simulink model "Feedback_NearestNeighbor"  (R2015a)
settings: Solver=ode3  StartTime=0.0  StopTime=500  FixedStep=0.01  MaxStep=0.01  RelTol=1e-3
values from neighbouring files (symbols this model uses):
  H0 = interp1q(Periodic_Solution(:,1),Periodic_Solution(:,4),Initial_Time-6)    [Feedback_Nearest_Neighbour_cross_validation.m]
  Imax = 10000    [Feedback_Nearest_Neighbour_cross_validation.m]
  n0 = interp1q(Periodic_Solution(:,1),Periodic_Solution(:,7),Initial_Time-6)    [Feedback_Nearest_Neighbour_cross_validation.m]
  Periodic_Solution = Periodic_Solution(N:end,:)    [Feedback_Nearest_Neighbour_cross_validation.m]
  Sleep0 = interp1q(Periodic_Solution(:,1),Periodic_Solution(:,6),Initial_Time-6)    [Feedback_Nearest_Neighbour_cross_validation.m]
  tol = 0.01    [Feedback_Nearest_Neighbour_cross_validation.m]
  x0 = interp1q(Periodic_Solution(:,1),Periodic_Solution(:,2),Initial_Time-6)    [Feedback_Nearest_Neighbour_cross_validation.m]
  xc0 = interp1q(Periodic_Solution(:,1),Periodic_Solution(:,3),Initial_Time-6)    [Feedback_Nearest_Neighbour_cross_validation.m]
undefined symbols (not defined in the file or in its folder): Train_Sleep, Train_Wake
settings Model: Creator=wangf7  LastModifiedBy=Jiawei Yin
settings OptimizationCC: ExpressionDepthLimit=2147483647
settings DebuggingCC: AlgebraicLoopMsg=none  ArtificialAlgebraicLoopMsg=none  UnderspecifiedInitializationDetection=Classic  MergeDetectMultiDrivingBlocksExec=none  SolverPrmCheckMsg=warning  StateNameClashWarn=warning

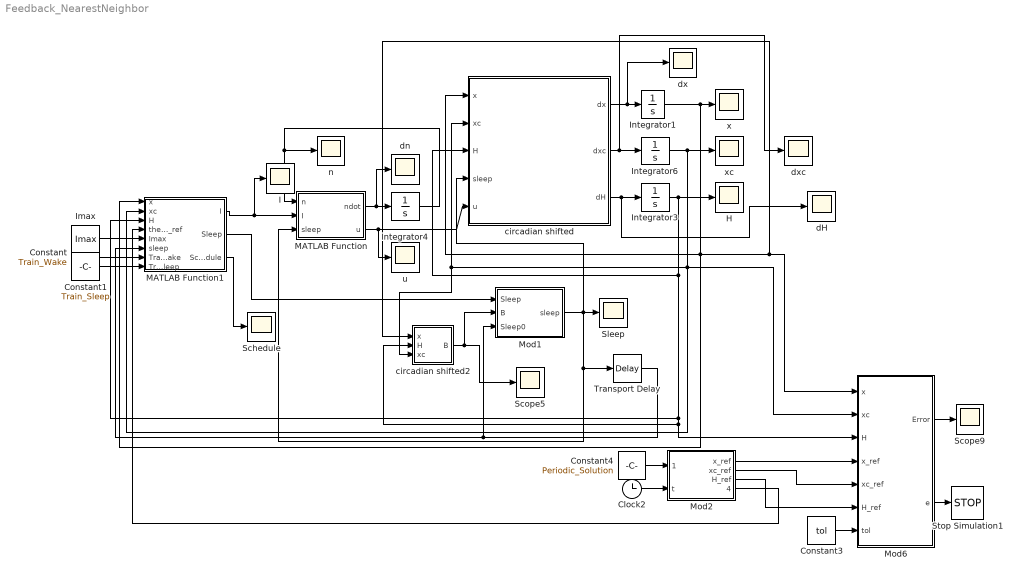
== system Feedback_NearestNeighbor ==
  Clock2 : Clock
  Constant : Constant  Value=Train_Wake
  Constant1 : Constant  Value=Train_Sleep
  Constant3 : Constant  Value=tol
  Constant4 : Constant  Value=Periodic_Solution
  H : Scope
      settings: TimeRange=auto  MaxDataPoints=5000  SaveName=H  YMin=-10  YMax=10  SampleTime=-1  DataFormat=Array
  I : Scope
      settings: TimeRange=auto  MaxDataPoints=5000  SaveName=I  YMin=-10  YMax=10  SampleTime=-1  DataFormat=Array
  Imax : Constant  Value=Imax
  Integrator1 : Integrator  InitialCondition=x0
  Integrator3 : Integrator  InitialCondition=H0
  Integrator4 : Integrator  InitialCondition=n0
  Integrator6 : Integrator  InitialCondition=xc0
  MATLAB Function : MATLAB Function  TreatAsAtomicUnit=on
      settings: PermitHierarchicalResolution=ParametersOnly
  MATLAB Function1 : MATLAB Function  TreatAsAtomicUnit=on
      settings: PermitHierarchicalResolution=ParametersOnly
  Mod1 : MATLAB Function  TreatAsAtomicUnit=on
      settings: PermitHierarchicalResolution=ParametersOnly
  Mod2 : MATLAB Function  TreatAsAtomicUnit=on
      settings: PermitHierarchicalResolution=ParametersOnly
  Mod6 : MATLAB Function  TreatAsAtomicUnit=on
      settings: PermitHierarchicalResolution=ParametersOnly
  Schedule : Scope
      settings: TimeRange=auto  MaxDataPoints=5000  SaveName=Schedule  YMin=-10  YMax=10  SampleTime=-1  DataFormat=Array
  Scope5 : Scope
      settings: TimeRange=auto  MaxDataPoints=5000  SaveName=B  YMin=-10  YMax=10  SampleTime=-1  DataFormat=Array
  Scope9 : Scope
      settings: TimeRange=auto  MaxDataPoints=5000  SaveName=Error  YMin=-10  YMax=10  SampleTime=-1  DataFormat=Array
  Sleep : Scope
      settings: TimeRange=auto  MaxDataPoints=5000  SaveName=Sleep  YMin=-10  YMax=10  SampleTime=-1  DataFormat=Array
  Stop Simulation1 : Stop
  Transport Delay : TransportDelay  DelayTime=.01  InitialOutput=Sleep0
  circadian shifted : MATLAB Function  TreatAsAtomicUnit=on
      settings: PermitHierarchicalResolution=ParametersOnly
  circadian shifted2 : MATLAB Function  TreatAsAtomicUnit=on
      settings: PermitHierarchicalResolution=ParametersOnly
  dH : Scope
      settings: TimeRange=auto  MaxDataPoints=5000  SaveName=dH  YMin=0.03966  YMax=0.05966  SampleTime=-1  DataFormat=Array
  dn : Scope
      settings: TimeRange=auto  MaxDataPoints=5000  SaveName=dn  YMin=-10  YMax=10  SampleTime=-1  DataFormat=Array
  dx : Scope
      settings: TimeRange=auto  MaxDataPoints=5000  SaveName=dx  YMin=-10  YMax=10  SampleTime=-1  DataFormat=Array
  dxc : Scope
      settings: TimeRange=auto  MaxDataPoints=5000  SaveName=dxc  YMin=-10  YMax=10  SampleTime=-1  DataFormat=Array
  n : Scope
      settings: TimeRange=auto  MaxDataPoints=5000  SaveName=n  YMin=-10  YMax=10  SampleTime=-1  DataFormat=Array
  u : Scope
      settings: TimeRange=auto  MaxDataPoints=5000  SaveName=u  YMin=-10  YMax=10  SampleTime=-1  DataFormat=Array
  x : Scope
      settings: TimeRange=auto  MaxDataPoints=5000  SaveName=x  YMin=-10  YMax=10  SampleTime=-1  DataFormat=Array
  xc : Scope
      settings: TimeRange=auto  MaxDataPoints=5000  SaveName=xc  YMin=-10  YMax=10  SampleTime=-1  DataFormat=Array
  wires:
  circadian shifted/1(dx) -> Integrator1/1, dx/1
  Integrator1/1 -> MATLAB Function1/1(x), circadian shifted2/1(x), Mod6/1(x), circadian shifted/1(x), x/1
  Integrator6/1 -> MATLAB Function1/2(xc), Mod6/2(xc), circadian shifted/2(xc), circadian shifted2/3(xc), xc/1
  circadian shifted2/1(B) -> Scope5/1, Mod1/2(B)
  Mod1/1(sleep) -> MATLAB Function/3(sleep), Transport Delay/1, Sleep/1, circadian shifted/4(sleep)
  Constant4/1 -> Mod2/1(Periodic_Solution)
  Clock2/1 -> Mod2/2(t)
  Mod6/2(e) -> Stop Simulation1/1
  Mod6/1(Error) -> Scope9/1
  Mod2/3(H_ref) -> Mod6/6(H_ref)
  Constant3/1 -> Mod6/7(tol)
  circadian shifted/2(dxc) -> Integrator6/1, dxc/1
  Integrator3/1 -> MATLAB Function1/3(H), circadian shifted2/2(H), Mod6/3(H), circadian shifted/3(H), H/1
  Mod2/1(x_ref) -> Mod6/4(x_ref)
  Mod2/2(xc_ref) -> Mod6/5(xc_ref)
  circadian shifted/3(dH) -> dH/1, Integrator3/1
  MATLAB Function/2(u) -> u/1, circadian shifted/5(u)
  MATLAB Function/1(ndot) -> dn/1, Integrator4/1
  Integrator4/1 -> n/1, MATLAB Function/1(n)
  MATLAB Function1/1(I) -> I/1, MATLAB Function/2(I)
  Constant/1 -> MATLAB Function1/7(Train_Wake)
  Mod2/4(theta_ref) -> MATLAB Function1/4(theta_ref)
  Imax/1 -> MATLAB Function1/5(Imax)
  MATLAB Function1/2(Sleep) -> Mod1/1(Sleep)
  Transport Delay/1 -> MATLAB Function1/6(sleep), Mod1/3(Sleep0)
  MATLAB Function1/3(Schedule) -> Schedule/1
  Constant1/1 -> MATLAB Function1/8(Train_Sleep)

== matlab function Feedback_NearestNeighbor/MATLAB Function1 ==
  data: x input; xc input; H input; theta_ref input; Imax input; sleep input; Train_Wake input; I output; Sleep output; Schedule output; Train_Sleep input
function [I,Sleep,Schedule] = fcn(x,xc,H,theta_ref,Imax,sleep,Train_Wake,Train_Sleep)
Idx=0;
coder.extrinsic('dsearchn')
if sleep==0
    Idx=dsearchn(Train_Wake(:,1:3),[mod(atan2(-xc,x),2*pi),H,theta_ref]);
    II=Train_Wake(Idx,5);
    if II>Imax/2
        I=Imax;
    else
        I=0;
    end
    Schedule=Train_Wake(Idx,6);
    if Schedule<=0.01
        Sleep=1;
    else
        Sleep=0;
    end
else
    Idx=dsearchn(Train_Sleep(:,1:3),[mod(atan2(-xc,x),2*pi),H,theta_ref]);
    Schedule=Train_Sleep(Idx,6);
    I=0;
    if Schedule<=0.01
        Sleep=0;
    else
        Sleep=1;
    end
end

== matlab function Feedback_NearestNeighbor/Mod1 ==
  data: Sleep input; sleep output; B input; Sleep0 input
function sleep = fcn(Sleep,B,Sleep0)
%#codegen
sleep=round(Sleep);

if sleep==0 && round(Sleep0)==1
    if B>0.27
        sleep=1;
    end 
elseif sleep==1 && round(Sleep0)==0
    if B<0.67
        sleep=0;
    end
end

if B>0.77
    sleep=1;
elseif B<0.17
    sleep=0;
end

== matlab function Feedback_NearestNeighbor/MATLAB Function ==
  data: n input; I input; ndot output; u output; sleep input
function [ndot,u] = fcn(n,I,sleep)
G=33.75;
alpha0=0.05;
beta=0.0075;
I0=9500;
alpha=alpha0*(I*(1-sleep)/I0)^0.5;
u=G*alpha*(1-n);
ndot=60*[alpha*(1-n)-beta*n];

== matlab function Feedback_NearestNeighbor/circadian shifted ==
  data: x input; xc input; H input; sleep input; u input; dx output; dxc output; dH output
function [dx,dxc,dH] = fcn(x,xc,H,sleep,u)
%#eml

tr=18.2;
td=4.2;

q = 1/3;
taux = 24.2;
k = 0.55;
mu=0.13;

B = u*(1-0.4*x)*(1-0.4*xc)*(1-sleep);

dx = (pi/12)*(xc + B  + mu*(1/3*x + 4/3*x^3 - 256/105*x^7));
dxc = (pi/12)*(q*B *xc - (24/(taux*0.99729))^2*x - k*B*x);
dH = (1-sleep)*(1-H)/tr-(H*sleep)/td;

== matlab function Feedback_NearestNeighbor/circadian shifted2 ==
  data: x input; H input; B output; xc input
function B = fcn(x,H,xc)
%#eml
B=H-0.1333*x;

== matlab function Feedback_NearestNeighbor/Mod2 ==
  data: Periodic_Solution input; x_ref output; xc_ref output; t input; H_ref output; theta_ref output
function [x_ref,xc_ref,H_ref,theta_ref] = fcn(Periodic_Solution,t)
%#codegen
x_ref=interp1q(Periodic_Solution(:,1),Periodic_Solution(:,2),t);
xc_ref=interp1q(Periodic_Solution(:,1),Periodic_Solution(:,3),t);
H_ref=interp1q(Periodic_Solution(:,1),Periodic_Solution(:,4),t);
theta_ref=mod(atan2(-xc_ref,x_ref),2*pi);

== matlab function Feedback_NearestNeighbor/Mod6 ==
  data: Error output; x input; xc input; H input; x_ref input; xc_ref input; e output; H_ref input; tol input
function [Error,e] = fcn(x,xc,H,x_ref,xc_ref,H_ref,tol)
%#codegen
Error=(H-H_ref)^2+(x-x_ref)^2+(xc-xc_ref)^2;
e=Error<tol;
